simulink model "lagrang"  (Simulink 7.9)
settings: Solver=ode45  StartTime=-10.0  StopTime=50.0  RelTol=1e-3
libraries: simulink x2
settings Model: Creator=Mihail  LastModifiedBy=Mihail

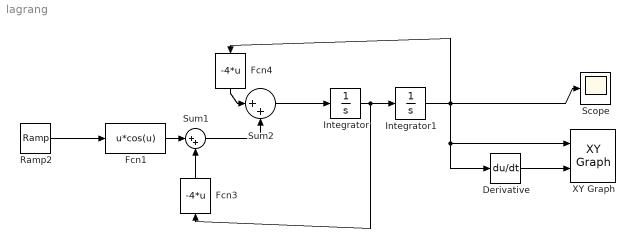
== system lagrang ==
  Derivative : Derivative
  Fcn1 : Fcn  Expr=u*cos(u)
  Fcn3 : Fcn  Expr=-4*u
  Fcn4 : Fcn  Expr=-4*u
  Integrator : Integrator
  Integrator1 : Integrator
  Ramp2 : simulink/Sources/Ramp  slope=1  start=1  X0=0
  Scope : Scope
      settings: YMin=6  YMax=10.25
  Sum1 : Sum  Inputs=|++
  Sum2 : Sum  Inputs=|++
  XY Graph : simulink/Sinks/XY Graph  xmin=-10  xmax=10  ymin=-10  ymax=10  st=0.01
  wires:
  Ramp2/1 -> Fcn1/1
  Integrator1/1 -> Derivative/1, XY Graph/1, Scope/1, Fcn4/1
  Integrator/1 -> Integrator1/1, Fcn3/1
  Sum2/1 -> Integrator/1
  Sum1/1 -> Sum2/2
  Fcn1/1 -> Sum1/1
  Derivative/1 -> XY Graph/2
  Fcn3/1 -> Sum1/2
  Fcn4/1 -> Sum2/1
